simulink model "AnalogEE_1s_1m"  (Simulink 7.5)
settings: Solver=ode45  StartTime=0.0  StopTime=3.0  RelTol=1e-3
libraries: NeuroModelerLibrary x6, simulink x2, neural x2
settings Model: Creator=user  LastModifiedBy=Bakhshiev
settings DebuggingCC: StrictBusMsg=Warning

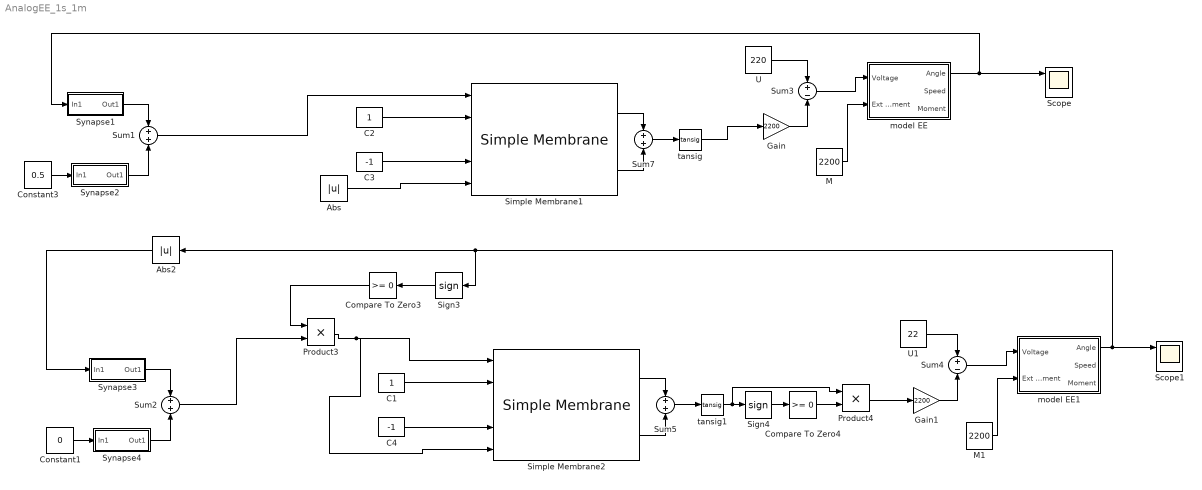
== system AnalogEE_1s_1m ==
  Abs : Abs  OutDataType=sfix(16)  OutScaling=2^0
  Abs2 : Abs  OutDataType=sfix(16)  OutScaling=2^0
  C1 : Constant  OutDataType=sfix(16)  OutScaling=2^0
  C2 : Constant  OutDataType=sfix(16)  OutScaling=2^0
  C3 : Constant  Value=-1  OutDataType=sfix(16)  OutScaling=2^0
  C4 : Constant  Value=-1  OutDataType=sfix(16)  OutScaling=2^0
  Compare To Zero3 : simulink/Logic and Bit Operations/Compare To Zero  SystemSampleTime=-1  relop=>=  LogicOutDataTypeMode=uint8  ZeroCross=off
  Compare To Zero4 : simulink/Logic and Bit Operations/Compare To Zero  SystemSampleTime=-1  relop=>=  LogicOutDataTypeMode=uint8  ZeroCross=off
  Constant1 : Constant  Value=0  OutDataType=sfix(16)  OutScaling=2^0
  Constant3 : Constant  Value=0.5  OutDataType=sfix(16)  OutScaling=2^0
  Gain : Gain  Gain=2200  ParameterDataType=sfix(16)  ParameterScaling=2^0  OutDataType=sfix(16)  OutScaling=2^0  SaturateOnIntegerOverflow=on  OutDataTypeStr=Inherit: Same as input  ParamDataTypeStr=Inherit: Same as input
  Gain1 : Gain  Gain=2200  ParameterDataType=sfix(16)  ParameterScaling=2^0  OutDataType=sfix(16)  OutScaling=2^0  SaturateOnIntegerOverflow=on  OutDataTypeStr=Inherit: Same as input  ParamDataTypeStr=Inherit: Same as input
  M : Constant  Value=2200  OutDataType=sfix(16)  OutScaling=2^0
  M1 : Constant  Value=2200  OutDataType=sfix(16)  OutScaling=2^0
  Product3 : Product  OutDataType=sfix(16)  OutScaling=2^0  RndMeth=Zero
  Product4 : Product  OutDataType=sfix(16)  OutScaling=2^0  RndMeth=Zero
  Scope : Scope  NumInputPorts=3
      settings: TimeRange=3  YMin=100~-1~-1  YMax=180~1~1
  Scope1 : Scope  NumInputPorts=3
      settings: TimeRange=3  YMin=-5~-1~-1  YMax=-2~1~1  SaveName=ScopeData2
  Sign3 : Signum
  Sign4 : Signum
  Simple Membrane1 : NeuroModelerLibrary/Neuron Elements/Simple Membrane  SystemSampleTime=-1  ACm=1e-9  ARm=1e7  ECm=1e-9  ERm=1e7  ARFm=1e8  ERFm=1e8
  Simple Membrane2 : NeuroModelerLibrary/Neuron Elements/Simple Membrane  SystemSampleTime=-1  ACm=1e-9  ARm=1e7  ECm=1e-9  ERm=1e7  ARFm=1e8  ERFm=1e8
  Sum{1..2,5,7} (4 alike) : Sum  OutDataType=sfix(16)  OutScaling=2^0  SaturateOnIntegerOverflow=on  InputSameDT=on  OutDataTypeStr=Inherit: Same as first input
  Sum3 : Sum  Inputs=+-  OutDataType=sfix(16)  OutScaling=2^0  SaturateOnIntegerOverflow=on  InputSameDT=on  OutDataTypeStr=Inherit: Same as first input
  Sum4 : Sum  Inputs=+-  OutDataType=sfix(16)  OutScaling=2^0  SaturateOnIntegerOverflow=on  InputSameDT=on  OutDataTypeStr=Inherit: Same as first input
  Synapse1 : Subsystem  AncestorBlock=NeuroModelerLibrary/Neuron Elements/Synapse  mask{SecretionTC=0.001, DecompositionTC=0.01, ksi=2, gamma=1e8}
      mask prompts: SecretionTC "Mediator Secretion"; DecompositionTC "Mediator Decomposition"
  Synapse2 : Subsystem  AncestorBlock=NeuroModelerLibrary/Neuron Elements/Synapse  mask{SecretionTC=0.001, DecompositionTC=0.01, ksi=2, gamma=1e8}
      mask prompts: SecretionTC "Mediator Secretion"; DecompositionTC "Mediator Decomposition"
  Synapse3 : Subsystem  AncestorBlock=NeuroModelerLibrary/Neuron Elements/Synapse  mask{SecretionTC=0.001, DecompositionTC=0.01, ksi=2, gamma=1e8}
      mask prompts: SecretionTC "Mediator Secretion"; DecompositionTC "Mediator Decomposition"
  Synapse4 : Subsystem  AncestorBlock=NeuroModelerLibrary/Neuron Elements/Synapse  mask{SecretionTC=0.001, DecompositionTC=0.01, ksi=2, gamma=1e8}
      mask prompts: SecretionTC "Mediator Secretion"; DecompositionTC "Mediator Decomposition"
  U : Constant  Value=220  OutDataType=sfix(16)  OutScaling=2^0
  U1 : Constant  Value=22  OutDataType=sfix(16)  OutScaling=2^0
  model EE : Subsystem
  model EE1 : Subsystem
  tansig : neural/Transfer Functions/tansig  SystemSampleTime=-1
  tansig1 : neural/Transfer Functions/tansig  SystemSampleTime=-1
  wires:
  C2/1 -> Simple Membrane1/2
  C3/1 -> Simple Membrane1/4
  Simple Membrane1/1 -> Sum7/1
  Simple Membrane1/2 -> Sum7/2
  Constant3/1 -> Synapse2/1(In1)
  Synapse1/1(Out1) -> Sum1/1
  Sum3/1 -> model EE/1(Voltage)
  Gain/1 -> Sum3/2
  U/1 -> Sum3/1
  M/1 -> model EE/2(Ext moment)
  model EE/1(Angle) -> Scope/1, Synapse1/1(In1)
  Abs/1 -> Simple Membrane1/5
  C1/1 -> Simple Membrane2/2
  C4/1 -> Simple Membrane2/4
  Simple Membrane2/1 -> Sum5/1
  Simple Membrane2/2 -> Sum5/2
  Sum5/1 -> tansig1/1
  Constant1/1 -> Synapse4/1(In1)
  Synapse3/1(Out1) -> Sum2/1
  Synapse4/1(Out1) -> Sum2/2
  Sum4/1 -> model EE1/1(Voltage)
  Gain1/1 -> Sum4/2
  U1/1 -> Sum4/1
  M1/1 -> model EE1/2(Ext moment)
  model EE1/1(Angle) -> Scope1/1, Abs2/1, Sign3/1
  Sign4/1 -> Compare To Zero4/1
  Compare To Zero4/1 -> Product4/2
  tansig1/1 -> Sign4/1, Product4/1
  Product4/1 -> Gain1/1
  Abs2/1 -> Synapse3/1(In1)
  Sign3/1 -> Compare To Zero3/1
  Compare To Zero3/1 -> Product3/1
  Sum2/1 -> Product3/2
  Product3/1 -> Simple Membrane2/1, Simple Membrane2/5
  Synapse2/1(Out1) -> Sum1/2
  Sum7/1 -> tansig/1
  tansig/1 -> Gain/1
  Sum1/1 -> Simple Membrane1/1

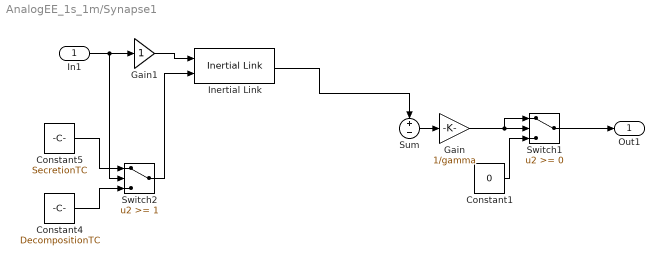
== system AnalogEE_1s_1m/Synapse1 ==
  In1 : Inport  OutDataType=sfix(16)  OutScaling=2^0
  Constant1 : Constant  Value=0  OutDataType=sfix(16)  OutScaling=2^0
  Constant4 : Constant  Value=DecompositionTC  OutDataType=sfix(16)  OutScaling=2^0
  Constant5 : Constant  Value=SecretionTC  OutDataType=sfix(16)  OutScaling=2^0
  Gain : Gain  Gain=1/gamma  ParameterDataType=sfix(16)  ParameterScaling=2^0  OutDataType=sfix(16)  OutScaling=2^0  SaturateOnIntegerOverflow=on  OutDataTypeStr=Inherit: Same as input  ParamDataTypeStr=Inherit: Same as input
  Gain1 : Gain  ParameterDataType=sfix(16)  ParameterScaling=2^0  OutDataType=sfix(16)  OutScaling=2^0  SaturateOnIntegerOverflow=on  OutDataTypeStr=Inherit: Same as input  ParamDataTypeStr=Inherit: Same as input
  Inertial Link : NeuroModelerLibrary/Support/Inertial Link  SystemSampleTime=-1
  Sum : Sum  Inputs=+-  OutDataType=sfix(16)  OutScaling=2^0  SaturateOnIntegerOverflow=on
  Switch1 : Switch
  Switch2 : Switch  Threshold=1
  Out1 : Outport  OutDataType=sfix(16)  OutScaling=2^0
  wires:
  Switch1/1 -> Out1/1
  Gain1/1 -> Inertial Link/1
  Constant1/1 -> Switch1/3
  Gain/1 -> Switch1/1, Switch1/2
  Switch2/1 -> Inertial Link/2
  Constant5/1 -> Switch2/1
  Constant4/1 -> Switch2/3
  Inertial Link/1 -> Sum/1
  Sum/1 -> Gain/1
  In1/1 -> Gain1/1, Switch2/2

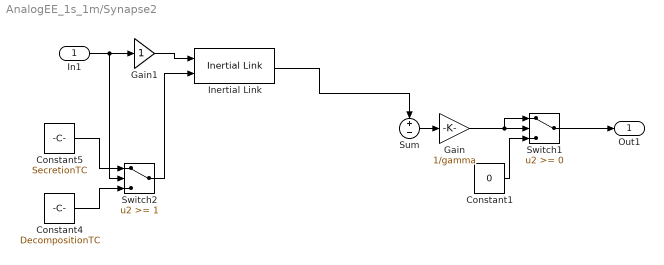
== system AnalogEE_1s_1m/Synapse2 ==
  In1 : Inport  OutDataType=sfix(16)  OutScaling=2^0
  Constant1 : Constant  Value=0  OutDataType=sfix(16)  OutScaling=2^0
  Constant4 : Constant  Value=DecompositionTC  OutDataType=sfix(16)  OutScaling=2^0
  Constant5 : Constant  Value=SecretionTC  OutDataType=sfix(16)  OutScaling=2^0
  Gain : Gain  Gain=1/gamma  ParameterDataType=sfix(16)  ParameterScaling=2^0  OutDataType=sfix(16)  OutScaling=2^0  SaturateOnIntegerOverflow=on  OutDataTypeStr=Inherit: Same as input  ParamDataTypeStr=Inherit: Same as input
  Gain1 : Gain  ParameterDataType=sfix(16)  ParameterScaling=2^0  OutDataType=sfix(16)  OutScaling=2^0  SaturateOnIntegerOverflow=on  OutDataTypeStr=Inherit: Same as input  ParamDataTypeStr=Inherit: Same as input
  Inertial Link : NeuroModelerLibrary/Support/Inertial Link  SystemSampleTime=-1
  Sum : Sum  Inputs=+-  OutDataType=sfix(16)  OutScaling=2^0  SaturateOnIntegerOverflow=on
  Switch1 : Switch
  Switch2 : Switch  Threshold=1
  Out1 : Outport  OutDataType=sfix(16)  OutScaling=2^0
  wires:
  Switch1/1 -> Out1/1
  Gain1/1 -> Inertial Link/1
  Constant1/1 -> Switch1/3
  Gain/1 -> Switch1/1, Switch1/2
  Switch2/1 -> Inertial Link/2
  Constant5/1 -> Switch2/1
  Constant4/1 -> Switch2/3
  Inertial Link/1 -> Sum/1
  Sum/1 -> Gain/1
  In1/1 -> Gain1/1, Switch2/2

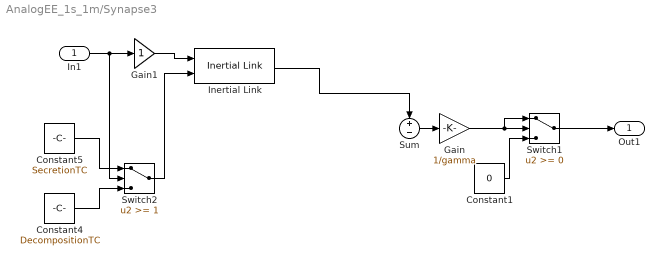
== system AnalogEE_1s_1m/Synapse3 ==
  In1 : Inport  OutDataType=sfix(16)  OutScaling=2^0
  Constant1 : Constant  Value=0  OutDataType=sfix(16)  OutScaling=2^0
  Constant4 : Constant  Value=DecompositionTC  OutDataType=sfix(16)  OutScaling=2^0
  Constant5 : Constant  Value=SecretionTC  OutDataType=sfix(16)  OutScaling=2^0
  Gain : Gain  Gain=1/gamma  ParameterDataType=sfix(16)  ParameterScaling=2^0  OutDataType=sfix(16)  OutScaling=2^0  SaturateOnIntegerOverflow=on  OutDataTypeStr=Inherit: Same as input  ParamDataTypeStr=Inherit: Same as input
  Gain1 : Gain  ParameterDataType=sfix(16)  ParameterScaling=2^0  OutDataType=sfix(16)  OutScaling=2^0  SaturateOnIntegerOverflow=on  OutDataTypeStr=Inherit: Same as input  ParamDataTypeStr=Inherit: Same as input
  Inertial Link : NeuroModelerLibrary/Support/Inertial Link  SystemSampleTime=-1
  Sum : Sum  Inputs=+-  OutDataType=sfix(16)  OutScaling=2^0  SaturateOnIntegerOverflow=on
  Switch1 : Switch
  Switch2 : Switch  Threshold=1
  Out1 : Outport  OutDataType=sfix(16)  OutScaling=2^0
  wires:
  Switch1/1 -> Out1/1
  Gain1/1 -> Inertial Link/1
  Constant1/1 -> Switch1/3
  Gain/1 -> Switch1/1, Switch1/2
  Switch2/1 -> Inertial Link/2
  Constant5/1 -> Switch2/1
  Constant4/1 -> Switch2/3
  Inertial Link/1 -> Sum/1
  Sum/1 -> Gain/1
  In1/1 -> Gain1/1, Switch2/2

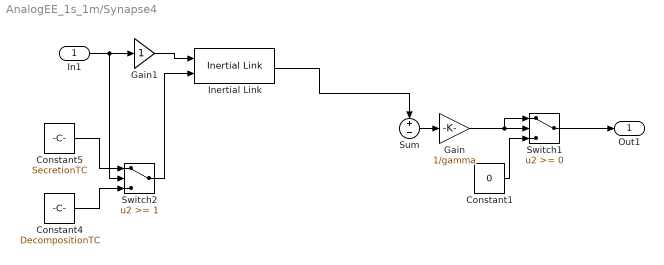
== system AnalogEE_1s_1m/Synapse4 ==
  In1 : Inport  OutDataType=sfix(16)  OutScaling=2^0
  Constant1 : Constant  Value=0  OutDataType=sfix(16)  OutScaling=2^0
  Constant4 : Constant  Value=DecompositionTC  OutDataType=sfix(16)  OutScaling=2^0
  Constant5 : Constant  Value=SecretionTC  OutDataType=sfix(16)  OutScaling=2^0
  Gain : Gain  Gain=1/gamma  ParameterDataType=sfix(16)  ParameterScaling=2^0  OutDataType=sfix(16)  OutScaling=2^0  SaturateOnIntegerOverflow=on  OutDataTypeStr=Inherit: Same as input  ParamDataTypeStr=Inherit: Same as input
  Gain1 : Gain  ParameterDataType=sfix(16)  ParameterScaling=2^0  OutDataType=sfix(16)  OutScaling=2^0  SaturateOnIntegerOverflow=on  OutDataTypeStr=Inherit: Same as input  ParamDataTypeStr=Inherit: Same as input
  Inertial Link : NeuroModelerLibrary/Support/Inertial Link  SystemSampleTime=-1
  Sum : Sum  Inputs=+-  OutDataType=sfix(16)  OutScaling=2^0  SaturateOnIntegerOverflow=on
  Switch1 : Switch
  Switch2 : Switch  Threshold=1
  Out1 : Outport  OutDataType=sfix(16)  OutScaling=2^0
  wires:
  Switch1/1 -> Out1/1
  Gain1/1 -> Inertial Link/1
  Constant1/1 -> Switch1/3
  Gain/1 -> Switch1/1, Switch1/2
  Switch2/1 -> Inertial Link/2
  Constant5/1 -> Switch2/1
  Constant4/1 -> Switch2/3
  Inertial Link/1 -> Sum/1
  Sum/1 -> Gain/1
  In1/1 -> Gain1/1, Switch2/2

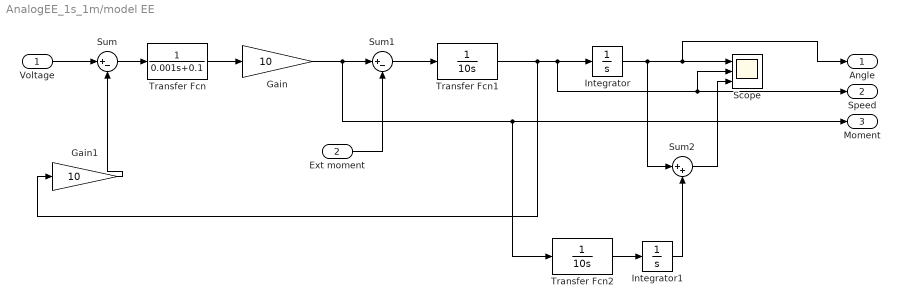
== system AnalogEE_1s_1m/model EE ==
  Voltage : Inport
  Ext moment : Inport  Port=2
  Gain : Gain  Gain=10
  Gain1 : Gain  Gain=10
  Integrator : Integrator
  Integrator1 : Integrator
  Scope : Scope  NumInputPorts=3
      settings: YMin=-700000~-4.5e+008~-1.5e+006  YMax=100000~5e+007~250000
  Sum : Sum  Inputs=|+-
  Sum1 : Sum  Inputs=|+-
  Sum2 : Sum  Inputs=|++
  Transfer Fcn : TransferFcn  Denominator=[0.001 0.1]
  Transfer Fcn1 : TransferFcn  Denominator=[10 0]
  Transfer Fcn2 : TransferFcn  Denominator=[10 0]
  Angle : Outport  Tag=Angle
  Speed : Outport  Port=2
  Moment : Outport  Port=3
  wires:
  Voltage/1 -> Sum/1
  Sum/1 -> Transfer Fcn/1
  Transfer Fcn/1 -> Gain/1
  Gain/1 -> Sum1/1, Transfer Fcn2/1, Moment/1
  Sum1/1 -> Transfer Fcn1/1
  Transfer Fcn1/1 -> Integrator/1, Scope/2, Speed/1, Gain1/1
  Gain1/1 -> Sum/2
  Ext moment/1 -> Sum1/2
  Integrator/1 -> Angle/1, Scope/1, Sum2/1
  Transfer Fcn2/1 -> Integrator1/1
  Integrator1/1 -> Sum2/2
  Sum2/1 -> Scope/3

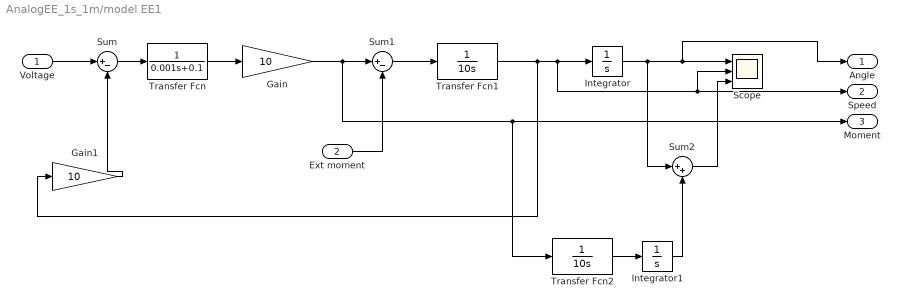
== system AnalogEE_1s_1m/model EE1 ==
  Voltage : Inport
  Ext moment : Inport  Port=2
  Gain : Gain  Gain=10
  Gain1 : Gain  Gain=10
  Integrator : Integrator
  Integrator1 : Integrator
  Scope : Scope  NumInputPorts=3
      settings: YMin=-700000~-4.5e+008~-1.5e+006  YMax=100000~5e+007~250000
  Sum : Sum  Inputs=|+-
  Sum1 : Sum  Inputs=|+-
  Sum2 : Sum  Inputs=|++
  Transfer Fcn : TransferFcn  Denominator=[0.001 0.1]
  Transfer Fcn1 : TransferFcn  Denominator=[10 0]
  Transfer Fcn2 : TransferFcn  Denominator=[10 0]
  Angle : Outport  Tag=Angle
  Speed : Outport  Port=2
  Moment : Outport  Port=3
  wires:
  Voltage/1 -> Sum/1
  Sum/1 -> Transfer Fcn/1
  Transfer Fcn/1 -> Gain/1
  Gain/1 -> Sum1/1, Transfer Fcn2/1, Moment/1
  Sum1/1 -> Transfer Fcn1/1
  Transfer Fcn1/1 -> Integrator/1, Scope/2, Speed/1, Gain1/1
  Gain1/1 -> Sum/2
  Ext moment/1 -> Sum1/2
  Integrator/1 -> Angle/1, Scope/1, Sum2/1
  Transfer Fcn2/1 -> Integrator1/1
  Integrator1/1 -> Sum2/2
  Sum2/1 -> Scope/3
